simulink model "Multi_Agent_Problem"  (R2022a)
settings: Solver=ode45  StartTime=0.0  StopTime=20  RelTol=1e-3
values from neighbouring files (symbols this model uses):
  B1_inv = B1_inv(:,2)    [Dynamic_Inversion.m]    (also in Linear_Model.mat = [0.0377096774194 0 -0.0377096774194 0])
  B2_inv = B2_inv(:,2)    [Dynamic_Inversion.m]    (also in Linear_Model.mat = [0 -0.0371290322581 0 0.0371290322581])
  B3_inv = B3_inv(:,1)    [Dynamic_Inversion.m]    (also in Linear_Model.mat = [0.0031875 -0.0031875 0.0031875 -0.0031875])
  B4_inv = pinv(B4)    [Dynamic_Inversion.m]    (also in Linear_Model.mat = [-0.25 -0.25 -0.25 -0.25])
  eta = 1    [Properties_Quad.m]
  g = 9.8    [Properties_Quad.m]
  L = 0.155    [Properties_Quad.m]
  m = 4    [Controller_LQR.m]    (also in Properties_Quad.m = 1)
  mass = 0.9    [Properties_Quad.m]
  r = [ones(1,length(t))]    [Hinf_Controller_Create.m]    (also in Properties_Quad.m = 1.5)
  u_e = zeros(4,1)    [Controller_LQR.m]    (also in Dynamic_Inversion.m; Linear_Model.mat = [2.45 2.45 2.45 2.45])
  w1_in = 4    [Dynamic_Inversion.m]    (also in Linear_Model.mat)
  w1_out = 1    [Dynamic_Inversion.m]    (also in Linear_Model.mat)
  w2_in = 4    [Dynamic_Inversion.m]    (also in Linear_Model.mat)
  w2_out = 1    [Dynamic_Inversion.m]    (also in Linear_Model.mat)
  w3_in = 4    [Dynamic_Inversion.m]    (also in Linear_Model.mat)
  w4_in = 3    [Dynamic_Inversion.m]    (also in Linear_Model.mat)
  zeta1_in = 0.7    [Dynamic_Inversion.m]    (also in Linear_Model.mat)
  zeta1_out = 0.7    [Dynamic_Inversion.m]    (also in Linear_Model.mat)
  zeta2_in = 0.7    [Dynamic_Inversion.m]    (also in Linear_Model.mat)
  zeta2_out = 0.7    [Dynamic_Inversion.m]    (also in Linear_Model.mat)
  zeta3_in = 0.7    [Dynamic_Inversion.m]    (also in Linear_Model.mat)
  zeta4_in = 0.7    [Dynamic_Inversion.m]    (also in Linear_Model.mat)
undefined symbols (not defined in the file or in its folder): magnitude
libraries: aerolibutil x4, rllib x3, shared6dof x3
(part 1 of 2)
settings Model: Creator=vicen  LastModifiedBy=vicen
settings DebuggingCC: UnconnectedInputMsg=warning  UnconnectedOutputMsg=warning  UnconnectedLineMsg=warning
settings RTWCC: DLArmComputeVersion=19.05

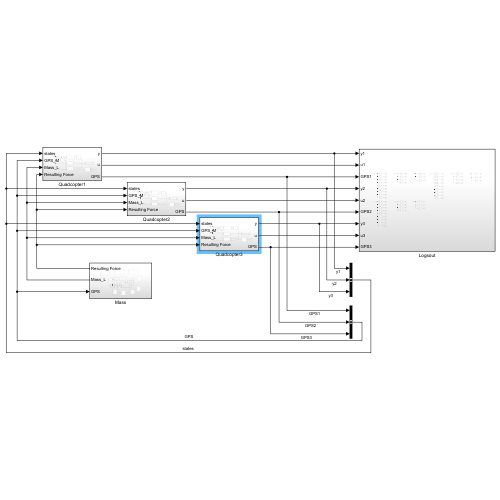
[thumbnail: Simulink's stored preview of the top-level diagram]
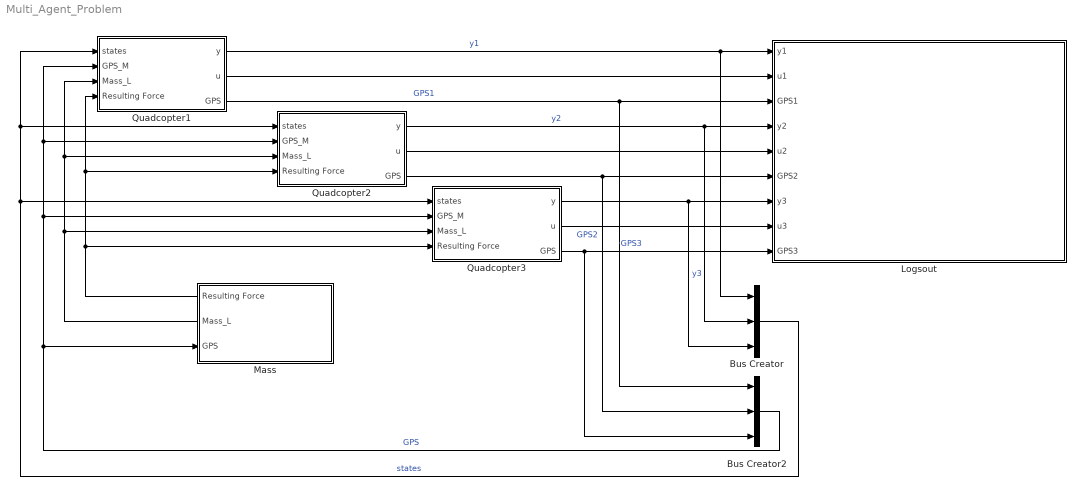
== system Multi_Agent_Problem ==
  Bus Creator : BusCreator  Inputs=3
  Bus Creator2 : BusCreator  Inputs=3
  Logsout : Subsystem
  Mass : Subsystem
      settings: PortSchema="{\"entries\":[{\"content\":{\"sides\":[{\"content\":{\"connectorIds\":[\"Out1\",\"Out2\",\"In1\"]},\"type\":\"ConnectorPlacement.EquallySpacedRectSide\",\"uuid\":\"4edc069a-805e-4b8f-97a6-cf234fccdbf6\"},{\"content\":{\"connectorIds\":[],\"side\":\"RIGHT\"},\"type\":\"ConnectorPlacement.EquallySpacedRectSide\",\"uuid\":\"8a591d16-4bf7-485b-b559-b7d05b260f63\"},{\"content\":{\"connectorIds\":[],\"side\":\"TOP\"},\"type\":\"ConnectorPlacement.EquallySpacedRectSide\",\"uuid\":\"cabdf924-e171-4e83-9a3e-1a1cf6358306\"},{\"content\":{\"connectorIds\":[],\"side\":\"BOTTOM\"},\"type\":\"ConnectorPlacement.EquallySpacedRectSide\",\"uuid\":\"5e829002-7c81-40d6-aefe-71acdfd17489\"}]},\"type\":\"ConnectorPlacement.EquallySpacedConnector\",\"uuid\":\"c7584162-5ecb-4d0e-90b3-ad9ea7690d4d\"}],\"packageUris\":[\"http://schema.mathworks.com/mf0/Connector/R2020b\"],\"version\":\"1.0\"}"
  Quadcopter1 : Subsystem
  Quadcopter2 : Subsystem
  Quadcopter3 : Subsystem
  wires:
  Quadcopter1/1(y) -> Logsout/1(y1), Bus Creator/1  "y1"
  Quadcopter1/2(u) -> Logsout/2(u1)
  Quadcopter1/3(GPS) -> Bus Creator2/1, Logsout/3(GPS1)  "GPS1"
  Quadcopter2/1(y) -> Logsout/4(y2), Bus Creator/2  "y2"
  Quadcopter2/2(u) -> Logsout/5(u2)
  Quadcopter2/3(GPS) -> Bus Creator2/2, Logsout/6(GPS2)  "GPS2"
  Quadcopter3/1(y) -> Logsout/7(y3), Bus Creator/3  "y3"
  Quadcopter3/2(u) -> Logsout/8(u3)
  Quadcopter3/3(GPS) -> Bus Creator2/3, Logsout/9(GPS3)  "GPS3"
  Bus Creator/1 -> Quadcopter3/1(states), Quadcopter2/1(states), Quadcopter1/1(states)  "states"
  Bus Creator2/1 -> Mass/1(GPS), Quadcopter3/2(GPS_M), Quadcopter2/2(GPS_M), Quadcopter1/2(GPS_M)  "GPS"
  Mass/1(Resulting Force) -> Quadcopter3/4("Resulting Force "), Quadcopter2/4("Resulting Force "), Quadcopter1/4("Resulting Force ")
  Mass/2(Mass_L) -> Quadcopter3/3(Mass_L), Quadcopter2/3(Mass_L), Quadcopter1/3(Mass_L)

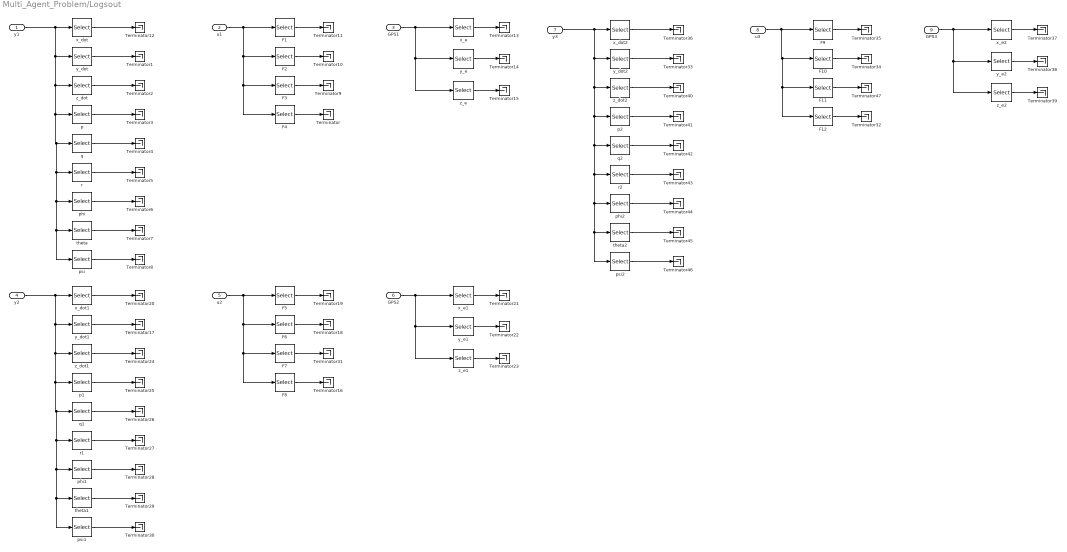
== system Multi_Agent_Problem/Logsout ==
  y1 : Inport
  u1 : Inport  Port=2
  GPS1 : Inport  Port=3
  y2 : Inport  Port=4
  u2 : Inport  Port=5
  GPS2 : Inport  Port=6
  y3 : Inport  Port=7
  u3 : Inport  Port=8
  GPS3 : Inport  Port=9
  F1 : Selector  InputPortWidth=4  IndexOptions=Index vector (dialog)  Indices=1  OutputSizes=1
  F10 : Selector  InputPortWidth=4  IndexOptions=Index vector (dialog)  Indices=2  OutputSizes=1
  F11 : Selector  InputPortWidth=4  IndexOptions=Index vector (dialog)  Indices=3  OutputSizes=1
  F12 : Selector  InputPortWidth=4  IndexOptions=Index vector (dialog)  Indices=4  OutputSizes=1
  F2 : Selector  InputPortWidth=4  IndexOptions=Index vector (dialog)  Indices=2  OutputSizes=1
  F3 : Selector  InputPortWidth=4  IndexOptions=Index vector (dialog)  Indices=3  OutputSizes=1
  F4 : Selector  InputPortWidth=4  IndexOptions=Index vector (dialog)  Indices=4  OutputSizes=1
  F5 : Selector  InputPortWidth=4  IndexOptions=Index vector (dialog)  Indices=1  OutputSizes=1
  F6 : Selector  InputPortWidth=4  IndexOptions=Index vector (dialog)  Indices=2  OutputSizes=1
  F7 : Selector  InputPortWidth=4  IndexOptions=Index vector (dialog)  Indices=3  OutputSizes=1
  F8 : Selector  InputPortWidth=4  IndexOptions=Index vector (dialog)  Indices=4  OutputSizes=1
  F9 : Selector  InputPortWidth=4  IndexOptions=Index vector (dialog)  Indices=1  OutputSizes=1
  Terminator{,1..47} (48 alike) : Terminator
  p : Selector  InputPortWidth=9  IndexOptions=Index vector (dialog)  Indices=4  OutputSizes=1
  p1 : Selector  InputPortWidth=9  IndexOptions=Index vector (dialog)  Indices=4  OutputSizes=1
  p2 : Selector  InputPortWidth=9  IndexOptions=Index vector (dialog)  Indices=4  OutputSizes=1
  phi : Selector  InputPortWidth=9  IndexOptions=Index vector (dialog)  Indices=7  OutputSizes=1
  phi1 : Selector  InputPortWidth=9  IndexOptions=Index vector (dialog)  Indices=7  OutputSizes=1
  phi2 : Selector  InputPortWidth=9  IndexOptions=Index vector (dialog)  Indices=7  OutputSizes=1
  psi : Selector  InputPortWidth=9  IndexOptions=Index vector (dialog)  Indices=9  OutputSizes=1
  psi1 : Selector  InputPortWidth=9  IndexOptions=Index vector (dialog)  Indices=9  OutputSizes=1
  psi2 : Selector  InputPortWidth=9  IndexOptions=Index vector (dialog)  Indices=9  OutputSizes=1
  q : Selector  InputPortWidth=9  IndexOptions=Index vector (dialog)  Indices=5  OutputSizes=1
  q1 : Selector  InputPortWidth=9  IndexOptions=Index vector (dialog)  Indices=5  OutputSizes=1
  q2 : Selector  InputPortWidth=9  IndexOptions=Index vector (dialog)  Indices=5  OutputSizes=1
  r : Selector  InputPortWidth=9  IndexOptions=Index vector (dialog)  Indices=6  OutputSizes=1
  r1 : Selector  InputPortWidth=9  IndexOptions=Index vector (dialog)  Indices=6  OutputSizes=1
  r2 : Selector  InputPortWidth=9  IndexOptions=Index vector (dialog)  Indices=6  OutputSizes=1
  theta : Selector  InputPortWidth=9  IndexOptions=Index vector (dialog)  Indices=8  OutputSizes=1
  theta1 : Selector  InputPortWidth=9  IndexOptions=Index vector (dialog)  Indices=8  OutputSizes=1
  theta2 : Selector  InputPortWidth=9  IndexOptions=Index vector (dialog)  Indices=8  OutputSizes=1
  x_dot : Selector  InputPortWidth=9  IndexOptions=Index vector (dialog)  Indices=1  OutputSizes=1
  x_dot1 : Selector  InputPortWidth=9  IndexOptions=Index vector (dialog)  Indices=1  OutputSizes=1
  x_dot2 : Selector  InputPortWidth=9  IndexOptions=Index vector (dialog)  Indices=1  OutputSizes=1
  x_e : Selector  InputPortWidth=3  IndexOptions=Index vector (dialog)  Indices=1  OutputSizes=1
  x_e1 : Selector  InputPortWidth=3  IndexOptions=Index vector (dialog)  Indices=1  OutputSizes=1
  x_e2 : Selector  InputPortWidth=3  IndexOptions=Index vector (dialog)  Indices=1  OutputSizes=1
  y_dot : Selector  InputPortWidth=9  IndexOptions=Index vector (dialog)  Indices=2  OutputSizes=1
  y_dot1 : Selector  InputPortWidth=9  IndexOptions=Index vector (dialog)  Indices=2  OutputSizes=1
  y_dot2 : Selector  InputPortWidth=9  IndexOptions=Index vector (dialog)  Indices=2  OutputSizes=1
  y_e : Selector  InputPortWidth=3  IndexOptions=Index vector (dialog)  Indices=2  OutputSizes=1
  y_e1 : Selector  InputPortWidth=3  IndexOptions=Index vector (dialog)  Indices=2  OutputSizes=1
  y_e2 : Selector  InputPortWidth=3  IndexOptions=Index vector (dialog)  Indices=2  OutputSizes=1
  z_dot : Selector  InputPortWidth=9  IndexOptions=Index vector (dialog)  Indices=3  OutputSizes=1
  z_dot1 : Selector  InputPortWidth=9  IndexOptions=Index vector (dialog)  Indices=3  OutputSizes=1
  z_dot2 : Selector  InputPortWidth=9  IndexOptions=Index vector (dialog)  Indices=3  OutputSizes=1
  z_e : Selector  InputPortWidth=3  IndexOptions=Index vector (dialog)  Indices=3  OutputSizes=1
  z_e1 : Selector  InputPortWidth=3  IndexOptions=Index vector (dialog)  Indices=3  OutputSizes=1
  z_e2 : Selector  InputPortWidth=3  IndexOptions=Index vector (dialog)  Indices=3  OutputSizes=1
  wires:
  y1/1 -> psi/1, theta/1, phi/1, r/1, q/1, p/1, z_dot/1, y_dot/1, x_dot/1
  x_dot/1 -> Terminator12/1
  y_dot/1 -> Terminator1/1
  z_dot/1 -> Terminator2/1
  p/1 -> Terminator3/1
  q/1 -> Terminator4/1
  r/1 -> Terminator5/1
  phi/1 -> Terminator6/1
  theta/1 -> Terminator7/1
  psi/1 -> Terminator8/1
  u1/1 -> F4/1, F3/1, F2/1, F1/1
  F1/1 -> Terminator11/1
  F2/1 -> Terminator10/1
  F3/1 -> Terminator9/1
  F4/1 -> Terminator/1
  GPS1/1 -> z_e/1, y_e/1, x_e/1
  x_e/1 -> Terminator13/1
  y_e/1 -> Terminator14/1
  z_e/1 -> Terminator15/1
  z_e1/1 -> Terminator23/1
  y_e1/1 -> Terminator22/1
  x_e1/1 -> Terminator21/1
  GPS2/1 -> x_e1/1, y_e1/1, z_e1/1
  F8/1 -> Terminator16/1
  F7/1 -> Terminator31/1
  F6/1 -> Terminator18/1
  F5/1 -> Terminator19/1
  u2/1 -> F5/1, F6/1, F7/1, F8/1
  psi1/1 -> Terminator30/1
  theta1/1 -> Terminator29/1
  phi1/1 -> Terminator28/1
  r1/1 -> Terminator27/1
  q1/1 -> Terminator26/1
  p1/1 -> Terminator25/1
  z_dot1/1 -> Terminator24/1
  y_dot1/1 -> Terminator17/1
  x_dot1/1 -> Terminator20/1
  y2/1 -> x_dot1/1, y_dot1/1, z_dot1/1, p1/1, q1/1, r1/1, phi1/1, theta1/1, psi1/1
  z_e2/1 -> Terminator39/1
  y_e2/1 -> Terminator38/1
  x_e2/1 -> Terminator37/1
  GPS3/1 -> x_e2/1, y_e2/1, z_e2/1
  F12/1 -> Terminator32/1
  F11/1 -> Terminator47/1
  F10/1 -> Terminator34/1
  F9/1 -> Terminator35/1
  u3/1 -> F9/1, F10/1, F11/1, F12/1
  psi2/1 -> Terminator46/1
  theta2/1 -> Terminator45/1
  phi2/1 -> Terminator44/1
  r2/1 -> Terminator43/1
  q2/1 -> Terminator42/1
  p2/1 -> Terminator41/1
  z_dot2/1 -> Terminator40/1
  y_dot2/1 -> Terminator33/1
  x_dot2/1 -> Terminator36/1
  y3/1 -> x_dot2/1, y_dot2/1, z_dot2/1, p2/1, q2/1, r2/1, phi2/1, theta2/1, psi2/1

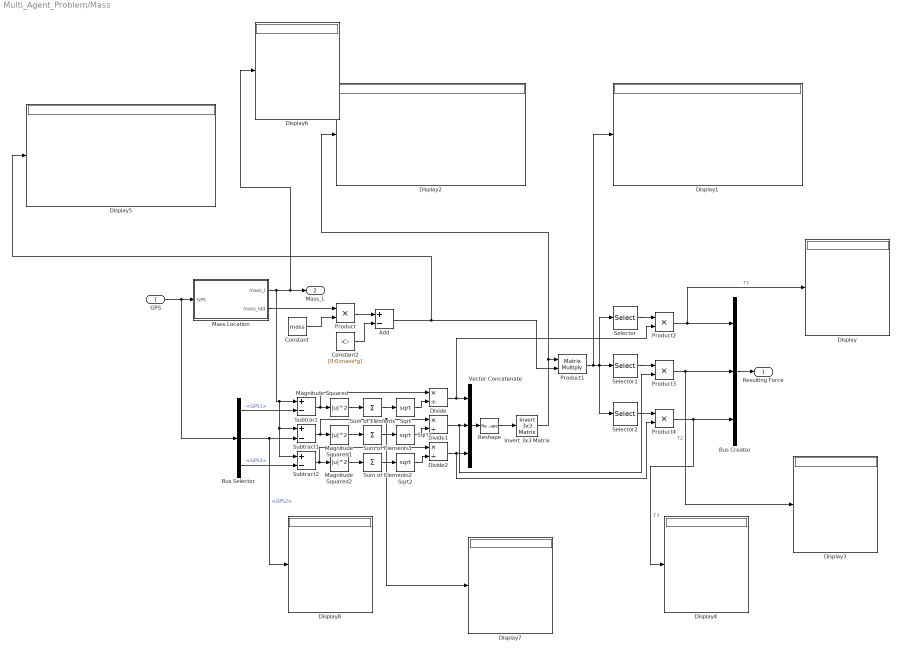
== system Multi_Agent_Problem/Mass ==
  GPS : Inport
  Add : Sum  Inputs=+-
  Bus Creator : BusCreator  Inputs=3
  Bus Selector : BusSelector  OutputSignals=GPS1,GPS2,GPS3
  Constant : Constant  Value=mass
  Constant2 : Constant  Value=[0;0;mass*g]
  Display{,1..8} (9 alike) : Display
  Divide : Product  Inputs=*/
  Divide1 : Product  Inputs=*/
  Divide2 : Product  Inputs=*/
  Invert 3x3 Matrix : aerolibutil/Invert  3x3 Matrix
  Magnitude Squared : Math  Operator=magnitude^2
  Magnitude Squared1 : Math  Operator=magnitude^2
  Magnitude Squared2 : Math  Operator=magnitude^2
  Mass Location : Subsystem
  Product{,2..4} (4 alike) : Product
  Product1 : Product  Multiplication=Matrix(*)
  Reshape : Reshape  OutputDimensionality=Customize  OutputDimensions=[3,3]
  Selector : Selector  InputPortWidth=3  IndexOptions=Index vector (dialog)  Indices=1  OutputSizes=1
  Selector1 : Selector  InputPortWidth=3  IndexOptions=Index vector (dialog)  Indices=2  OutputSizes=1
  Selector2 : Selector  InputPortWidth=3  IndexOptions=Index vector (dialog)  Indices=3  OutputSizes=1
  Sqrt : Sqrt
  Sqrt1 : Sqrt
  Sqrt2 : Sqrt
  Subtract : Sum  Inputs=+-
  Subtract1 : Sum  Inputs=+-
  Subtract2 : Sum  Inputs=+-
  Sum of Elements : Sum  Inputs=+
  Sum of Elements1 : Sum  Inputs=+
  Sum of Elements2 : Sum  Inputs=+
  Vector Concatenate : Concatenate  NumInputs=3
  Resulting Force : Outport
  Mass_L : Outport  Port=2
  wires:
  Constant/1 -> Product/2
  GPS/1 -> Bus Selector/1, Mass Location/1(GPS)
  Product/1 -> Add/1
  Constant2/1 -> Add/2
  Add/1 -> Display5/1, Product1/2
  Mass Location/2(mass_ldd) -> Product/1
  Bus Selector/1 -> Subtract/2  "<GPS1>"
  Bus Selector/2 -> Display8/1, Subtract1/2  "<GPS2>"
  Bus Selector/3 -> Subtract2/2  "<GPS3>"
  Magnitude Squared/1 -> Sum of Elements/1
  Sum of Elements/1 -> Sqrt/1
  Subtract/1 -> Divide/1, Magnitude Squared/1
  Sum of Elements1/1 -> Sqrt1/1
  Magnitude Squared1/1 -> Sum of Elements1/1
  Magnitude Squared2/1 -> Sum of Elements2/1
  Sum of Elements2/1 -> Sqrt2/1
  Subtract1/1 -> Display7/1, Divide1/1, Magnitude Squared1/1
  Subtract2/1 -> Divide2/1, Magnitude Squared2/1
  Sqrt/1 -> Divide/2
  Sqrt1/1 -> Divide1/2
  Sqrt2/1 -> Divide2/2
  Vector Concatenate/1 -> Reshape/1
  Reshape/1 -> Invert 3x3 Matrix/1
  Invert 3x3 Matrix/1 -> Display2/1, Product1/1
  Product1/1 -> Display1/1, Selector/1, Selector1/1, Selector2/1
  Selector/1 -> Product2/1
  Selector1/1 -> Product3/1
  Selector2/1 -> Product4/1
  Divide/1 -> Product2/2, Vector Concatenate/1
  Divide1/1 -> Vector Concatenate/2, Product3/2
  Divide2/1 -> Vector Concatenate/3, Product4/2
  Product2/1 -> Bus Creator/1, Display/1  "T1"
  Product3/1 -> Bus Creator/2, Display3/1  "T2"
  Product4/1 -> Bus Creator/3, Display4/1  "T3"
  Bus Creator/1 -> Resulting Force/1
  Mass Location/1(mass_l) -> Subtract1/1, Subtract2/1, Subtract/1, Display6/1, Mass_L/1

== system Multi_Agent_Problem/Quadcopter1 ==
  states : Inport
  GPS_M : Inport  Port=2
  Mass_L : Inport  Port=3
  "Resulting Force " : Inport  Port=4
  Add : Sum
  Bus Selector : BusSelector  OutputSignals=y,GPS
  Bus Selector1 : BusSelector  OutputSignals=T1
  Constant : Constant  Value=u_e
  Inner Loop Controller : Subsystem
      settings: PortSchema="{\"entries\":[{\"content\":{\"sides\":[{\"content\":{\"connectorIds\":[\"In1\"]},\"type\":\"ConnectorPlacement.EquallySpacedRectSide\",\"uuid\":\"666e7364-b111-4755-8f1d-083b40822e0a\"},{\"content\":{\"connectorIds\":[\"Out1\",\"In2\",\"In3\"],\"side\":\"RIGHT\"},\"type\":\"ConnectorPlacement.EquallySpacedRectSide\",\"uuid\":\"79960851-d5f8-4ed1-a120-baa8ff5c91cc\"},{\"content\":{\"connectorIds\":[],\"side\":\"TOP\"},\"type\":\"ConnectorPlacement.EquallySpacedRectSide\",\"uuid\":\"7e17e0c8-a495-4336-a986-2912f57e855c\"}]},\"type\":\"ConnectorPlacement.EquallySpacedConnector\",\"uuid\":\"73e8834a-8f7e-4b97-a075-5988e4100682\"}],\"packageUris\":[\"http://schema.mathworks.com/mf0/Connector/R2020b\"],\"version\":\"1.0\"}"
  Invert 3x3 Matrix : aerolibutil/Invert  3x3 Matrix
  Mission Planner : Subsystem
  Nonlinear System : Subsystem
      settings: PortSchema="{\"entries\":[{\"content\":{\"sides\":[{\"content\":{\"connectorIds\":[\"In1\",\"In2\",\"Out3\"]},\"type\":\"ConnectorPlacement.EquallySpacedRectSide\",\"uuid\":\"cab06217-b179-45bf-86f1-9cea28acaed0\"},{\"content\":{\"connectorIds\":[\"Out1\",\"Out2\"],\"side\":\"RIGHT\"},\"type\":\"ConnectorPlacement.EquallySpacedRectSide\",\"uuid\":\"5b831b23-67c9-4c45-aa0b-c8fd683f7f92\"},{\"content\":{\"connectorIds\":[],\"side\":\"TOP\"},\"type\":\"ConnectorPlacement.EquallySpacedRectSide\",\"uuid\":\"cc9770f4-03a0-4d6b-bae9-66d47aa444fc\"}]},\"type\":\"ConnectorPlacement.EquallySpacedConnector\",\"uuid\":\"fadffd99-ec6a-40bb-bf99-42c072ecc200\"}],\"packageUris\":[\"http://schema.mathworks.com/mf0/Connector/R2020b\"],\"version\":\"1.0\"}"
  Outer Loop Controller : Subsystem
      settings: PortSchema="{\"entries\":[{\"content\":{\"sides\":[{\"content\":{\"connectorIds\":[\"In1\",\"In2\"]},\"type\":\"ConnectorPlacement.EquallySpacedRectSide\",\"uuid\":\"0909ecc3-b9ee-46d0-b494-8211f486c818\"},{\"content\":{\"connectorIds\":[\"Out1\",\"In3\"],\"side\":\"RIGHT\"},\"type\":\"ConnectorPlacement.EquallySpacedRectSide\",\"uuid\":\"005e7a1d-8b7a-4f17-bab5-535ca2dfed14\"},{\"content\":{\"connectorIds\":[],\"side\":\"TOP\"},\"type\":\"ConnectorPlacement.EquallySpacedRectSide\",\"uuid\":\"0a4038b9-1305-4628-a808-cbdb517a3351\"}]},\"type\":\"ConnectorPlacement.EquallySpacedConnector\",\"uuid\":\"d0044b2e-92c2-4718-8256-3cc5618cd0b9\"}],\"packageUris\":[\"http://schema.mathworks.com/mf0/Connector/R2020b\"],\"version\":\"1.0\"}"
  Product : Product  Multiplication=Matrix(*)
  Sensors : Subsystem
  y : Outport
  u : Outport  Port=2
  GPS : Outport  Port=3
  wires:
  Nonlinear System/1(X_e) -> Sensors/1(X_e)
  Nonlinear System/2(x) -> Sensors/2(States)
  Sensors/1(Measured States) -> Inner Loop Controller/1(Measured States), Outer Loop Controller/1(Measured States), Bus Selector/1
  Outer Loop Controller/1(Outter Loop) -> Inner Loop Controller/3(Outter Loop)
  Bus Selector/2 -> GPS/1  "<GPS>"
  Bus Selector/1 -> y/1  "<y>"
  Mission Planner/1(Mission Planner) -> Outer Loop Controller/2(Mission Planner)
  Inner Loop Controller/1(u) -> Add/2
  Add/1 -> u/1, Nonlinear System/2(u)
  Constant/1 -> Add/1
  states/1 -> Mission Planner/2(states)
  GPS_M/1 -> Mission Planner/1(GPS)
  "Resulting Force "/1 -> Bus Selector1/1
  Mass_L/1 -> Mission Planner/3(Mass_L)
  Bus Selector1/1 -> Product/1, Nonlinear System/1(Resulting Force)  "<T1>"
  Nonlinear System/3(E2B) -> Invert 3x3 Matrix/1
  Invert 3x3 Matrix/1 -> Product/2
  Product/1 -> Outer Loop Controller/3(Tension Force), Inner Loop Controller/2(" Tension Force")

== system Multi_Agent_Problem/Quadcopter2 ==
  states : Inport
  GPS_M : Inport  Port=2
  Mass_L : Inport  Port=3
  "Resulting Force " : Inport  Port=4
  Add : Sum
  Bus Selector : BusSelector  OutputSignals=y,GPS
  Bus Selector1 : BusSelector  OutputSignals=T2
  Constant : Constant  Value=u_e
  Inner Loop Controller : Subsystem
      settings: PortSchema="{\"entries\":[{\"content\":{\"sides\":[{\"content\":{\"connectorIds\":[\"In1\"]},\"type\":\"ConnectorPlacement.EquallySpacedRectSide\",\"uuid\":\"666e7364-b111-4755-8f1d-083b40822e0a\"},{\"content\":{\"connectorIds\":[\"Out1\",\"In2\",\"In3\"],\"side\":\"RIGHT\"},\"type\":\"ConnectorPlacement.EquallySpacedRectSide\",\"uuid\":\"79960851-d5f8-4ed1-a120-baa8ff5c91cc\"},{\"content\":{\"connectorIds\":[],\"side\":\"TOP\"},\"type\":\"ConnectorPlacement.EquallySpacedRectSide\",\"uuid\":\"7e17e0c8-a495-4336-a986-2912f57e855c\"}]},\"type\":\"ConnectorPlacement.EquallySpacedConnector\",\"uuid\":\"73e8834a-8f7e-4b97-a075-5988e4100682\"}],\"packageUris\":[\"http://schema.mathworks.com/mf0/Connector/R2020b\"],\"version\":\"1.0\"}"
  Invert 3x3 Matrix : aerolibutil/Invert  3x3 Matrix
  Mission Planner : Subsystem
  Nonlinear System : Subsystem
      settings: PortSchema="{\"entries\":[{\"content\":{\"sides\":[{\"content\":{\"connectorIds\":[\"In1\",\"In2\",\"Out3\"]},\"type\":\"ConnectorPlacement.EquallySpacedRectSide\",\"uuid\":\"cab06217-b179-45bf-86f1-9cea28acaed0\"},{\"content\":{\"connectorIds\":[\"Out1\",\"Out2\"],\"side\":\"RIGHT\"},\"type\":\"ConnectorPlacement.EquallySpacedRectSide\",\"uuid\":\"5b831b23-67c9-4c45-aa0b-c8fd683f7f92\"},{\"content\":{\"connectorIds\":[],\"side\":\"TOP\"},\"type\":\"ConnectorPlacement.EquallySpacedRectSide\",\"uuid\":\"cc9770f4-03a0-4d6b-bae9-66d47aa444fc\"}]},\"type\":\"ConnectorPlacement.EquallySpacedConnector\",\"uuid\":\"fadffd99-ec6a-40bb-bf99-42c072ecc200\"}],\"packageUris\":[\"http://schema.mathworks.com/mf0/Connector/R2020b\"],\"version\":\"1.0\"}"
  Outer Loop Controller : Subsystem
      settings: PortSchema="{\"entries\":[{\"content\":{\"sides\":[{\"content\":{\"connectorIds\":[\"In1\",\"In2\"]},\"type\":\"ConnectorPlacement.EquallySpacedRectSide\",\"uuid\":\"0909ecc3-b9ee-46d0-b494-8211f486c818\"},{\"content\":{\"connectorIds\":[\"Out1\",\"In3\"],\"side\":\"RIGHT\"},\"type\":\"ConnectorPlacement.EquallySpacedRectSide\",\"uuid\":\"005e7a1d-8b7a-4f17-bab5-535ca2dfed14\"},{\"content\":{\"connectorIds\":[],\"side\":\"TOP\"},\"type\":\"ConnectorPlacement.EquallySpacedRectSide\",\"uuid\":\"0a4038b9-1305-4628-a808-cbdb517a3351\"}]},\"type\":\"ConnectorPlacement.EquallySpacedConnector\",\"uuid\":\"d0044b2e-92c2-4718-8256-3cc5618cd0b9\"}],\"packageUris\":[\"http://schema.mathworks.com/mf0/Connector/R2020b\"],\"version\":\"1.0\"}"
  Product : Product  Multiplication=Matrix(*)
  Sensors : Subsystem
  y : Outport
  u : Outport  Port=2
  GPS : Outport  Port=3
  wires:
  Mass_L/1 -> Mission Planner/3(Mass_L)
  "Resulting Force "/1 -> Bus Selector1/1
  GPS_M/1 -> Mission Planner/1(GPS)
  states/1 -> Mission Planner/2(states)
  Constant/1 -> Add/1
  Add/1 -> u/1, Nonlinear System/2(u)
  Inner Loop Controller/1(u) -> Add/2
  Mission Planner/1(Mission Planner) -> Outer Loop Controller/2(Mission Planner)
  Bus Selector/1 -> y/1  "<y>"
  Bus Selector/2 -> GPS/1  "<GPS>"
  Outer Loop Controller/1(Outter Loop) -> Inner Loop Controller/3(Outter Loop)
  Sensors/1(Measured States) -> Inner Loop Controller/1(Measured States), Outer Loop Controller/1(Measured States), Bus Selector/1
  Nonlinear System/2(x) -> Sensors/2(States)
  Nonlinear System/1(X_e) -> Sensors/1(X_e)
  Bus Selector1/1 -> Nonlinear System/1(Resulting Force), Product/1  "<T2>"
  Invert 3x3 Matrix/1 -> Product/2
  Product/1 -> Inner Loop Controller/2(Tension Force), Outer Loop Controller/3(Tension Force)
  Nonlinear System/3(E2B) -> Invert 3x3 Matrix/1

== system Multi_Agent_Problem/Quadcopter3 ==
  states : Inport
  GPS_M : Inport  Port=2
  Mass_L : Inport  Port=3
  "Resulting Force " : Inport  Port=4
  Add : Sum
  Bus Selector : BusSelector  OutputSignals=y,GPS
  Bus Selector1 : BusSelector  OutputSignals=T3
  Constant : Constant  Value=u_e
  Inner Loop Controller : Subsystem
      settings: PortSchema="{\"entries\":[{\"content\":{\"sides\":[{\"content\":{\"connectorIds\":[\"In1\"]},\"type\":\"ConnectorPlacement.EquallySpacedRectSide\",\"uuid\":\"666e7364-b111-4755-8f1d-083b40822e0a\"},{\"content\":{\"connectorIds\":[\"Out1\",\"In2\",\"In3\"],\"side\":\"RIGHT\"},\"type\":\"ConnectorPlacement.EquallySpacedRectSide\",\"uuid\":\"79960851-d5f8-4ed1-a120-baa8ff5c91cc\"},{\"content\":{\"connectorIds\":[],\"side\":\"TOP\"},\"type\":\"ConnectorPlacement.EquallySpacedRectSide\",\"uuid\":\"7e17e0c8-a495-4336-a986-2912f57e855c\"}]},\"type\":\"ConnectorPlacement.EquallySpacedConnector\",\"uuid\":\"73e8834a-8f7e-4b97-a075-5988e4100682\"}],\"packageUris\":[\"http://schema.mathworks.com/mf0/Connector/R2020b\"],\"version\":\"1.0\"}"
  Invert 3x3 Matrix : aerolibutil/Invert  3x3 Matrix
  Mission Planner : Subsystem
  Nonlinear System : Subsystem
      settings: PortSchema="{\"entries\":[{\"content\":{\"sides\":[{\"content\":{\"connectorIds\":[\"In1\",\"In2\",\"Out3\"]},\"type\":\"ConnectorPlacement.EquallySpacedRectSide\",\"uuid\":\"cab06217-b179-45bf-86f1-9cea28acaed0\"},{\"content\":{\"connectorIds\":[\"Out1\",\"Out2\"],\"side\":\"RIGHT\"},\"type\":\"ConnectorPlacement.EquallySpacedRectSide\",\"uuid\":\"5b831b23-67c9-4c45-aa0b-c8fd683f7f92\"},{\"content\":{\"connectorIds\":[],\"side\":\"TOP\"},\"type\":\"ConnectorPlacement.EquallySpacedRectSide\",\"uuid\":\"cc9770f4-03a0-4d6b-bae9-66d47aa444fc\"}]},\"type\":\"ConnectorPlacement.EquallySpacedConnector\",\"uuid\":\"fadffd99-ec6a-40bb-bf99-42c072ecc200\"}],\"packageUris\":[\"http://schema.mathworks.com/mf0/Connector/R2020b\"],\"version\":\"1.0\"}"
  Outer Loop Controller : Subsystem
      settings: PortSchema="{\"entries\":[{\"content\":{\"sides\":[{\"content\":{\"connectorIds\":[\"In1\",\"In2\"]},\"type\":\"ConnectorPlacement.EquallySpacedRectSide\",\"uuid\":\"0909ecc3-b9ee-46d0-b494-8211f486c818\"},{\"content\":{\"connectorIds\":[\"Out1\",\"In3\"],\"side\":\"RIGHT\"},\"type\":\"ConnectorPlacement.EquallySpacedRectSide\",\"uuid\":\"005e7a1d-8b7a-4f17-bab5-535ca2dfed14\"},{\"content\":{\"connectorIds\":[],\"side\":\"TOP\"},\"type\":\"ConnectorPlacement.EquallySpacedRectSide\",\"uuid\":\"0a4038b9-1305-4628-a808-cbdb517a3351\"}]},\"type\":\"ConnectorPlacement.EquallySpacedConnector\",\"uuid\":\"d0044b2e-92c2-4718-8256-3cc5618cd0b9\"}],\"packageUris\":[\"http://schema.mathworks.com/mf0/Connector/R2020b\"],\"version\":\"1.0\"}"
  Product : Product  Multiplication=Matrix(*)
  Sensors : Subsystem
  y : Outport
  u : Outport  Port=2
  GPS : Outport  Port=3
  wires:
  Nonlinear System/1(X_e) -> Sensors/1(X_e)
  Nonlinear System/2(x) -> Sensors/2(States)
  Sensors/1(Measured States) -> Bus Selector/1, Outer Loop Controller/1(Measured States), Inner Loop Controller/1(Measured States)
  Outer Loop Controller/1(Outter Loop) -> Inner Loop Controller/3(Outter Loop)
  Bus Selector/2 -> GPS/1  "<GPS>"
  Bus Selector/1 -> y/1  "<y>"
  Mission Planner/1(Mission Planner) -> Outer Loop Controller/2(Mission Planner)
  Inner Loop Controller/1(u) -> Add/2
  Add/1 -> u/1, Nonlinear System/2(u)
  Constant/1 -> Add/1
  states/1 -> Mission Planner/2(states)
  GPS_M/1 -> Mission Planner/1(GPS)
  "Resulting Force "/1 -> Bus Selector1/1
  Mass_L/1 -> Mission Planner/3(Mass_L)
  Bus Selector1/1 -> Nonlinear System/1(Resulting Force), Product/1  "<T3>"
  Invert 3x3 Matrix/1 -> Product/2
  Product/1 -> Outer Loop Controller/3(Tension Force), Inner Loop Controller/2(Tension Force)
  Nonlinear System/3(E2B) -> Invert 3x3 Matrix/1

== system Multi_Agent_Problem/Mass/Mass Location ==
  GPS : Inport
  Bus Selector : BusSelector  OutputSignals=GPS1,GPS2,GPS3
  Constant : Constant  Value=r
  Derivative : Derivative
  Derivative1 : Derivative
  Display{,1..4} (5 alike) : Display
  Mass Location : MATLAB Function  TreatAsAtomicUnit=on
  mass_l : Outport
  mass_ldd : Outport  Port=2
  wires:
  Constant/1 -> Display4/1, Mass Location/4(r)
  Bus Selector/3 -> Mass Location/3(P3), Display3/1  "<GPS3>"
  Bus Selector/2 -> Mass Location/2(P2), Display2/1  "<GPS2>"
  Bus Selector/1 -> Display1/1, Mass Location/1(P1)  "<GPS1>"
  GPS/1 -> Bus Selector/1
  Derivative/1 -> mass_ldd/1
  Mass Location/1(mass_l) -> Display/1, mass_l/1, Derivative1/1
  Derivative1/1 -> Derivative/1

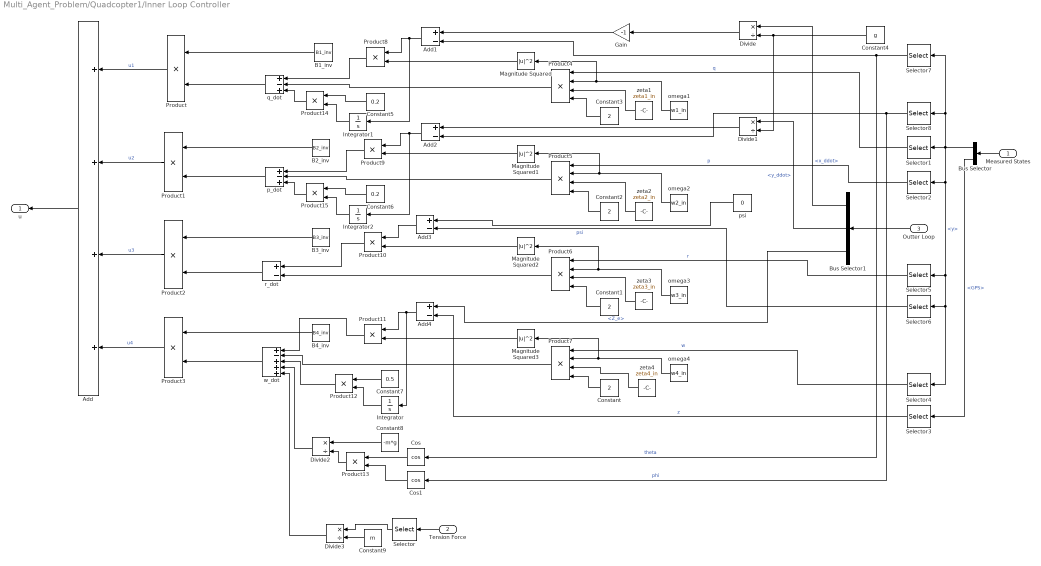
== system Multi_Agent_Problem/Quadcopter1/Inner Loop Controller ==
  Measured States : Inport
  " Tension Force" : Inport  Port=2
  Outter Loop : Inport  Port=3
  Add : Sum  Inputs=++++
  Add{1..4} (4 alike) : Sum  Inputs=+-
  B1_inv : Constant  Value=B1_inv
  B2_inv : Constant  Value=B2_inv
  B3_inv : Constant  Value=B3_inv
  B4_inv : Constant  Value=B4_inv
  Bus Selector : BusSelector  OutputSignals=y,GPS
  Bus Selector1 : BusSelector  OutputSignals=x_ddot,y_ddot,Z_e
  Constant{,1..3} (4 alike) : Constant  Value=2
  Constant4 : Constant  Value=g
  Constant5 : Constant  Value=0.2
  Constant6 : Constant  Value=0.2
  Constant7 : Constant  Value=0.5
  Constant8 : Constant  Value=-m*g
  Constant9 : Constant  Value=m
  Cos : Trigonometry  Operator=cos
  Cos1 : Trigonometry  Operator=cos
  Divide{,1..3} (4 alike) : Product  Inputs=*/
  Gain : Gain  Gain=-1
  Integrator : Integrator
  Integrator1 : Integrator
  Integrator2 : Integrator
  Magnitude Squared{,1..3} (4 alike) : Math  Operator=magnitude^2
  Product{,1..3,8..15} (12 alike) : Product
  Product{4..7} (4 alike) : Product  Inputs=4
  Selector : Selector  InputPortWidth=3  IndexOptions=Index vector (dialog)  Indices=3  OutputSizes=1
  Selector1 : Selector  InputPortWidth=9  IndexOptions=Index vector (dialog)  Indices=5  OutputSizes=1
  Selector2 : Selector  InputPortWidth=9  IndexOptions=Index vector (dialog)  Indices=4  OutputSizes=1
  Selector3 : Selector  InputPortWidth=3  IndexOptions=Index vector (dialog)  Indices=3  OutputSizes=1
  Selector4 : Selector  InputPortWidth=9  IndexOptions=Index vector (dialog)  Indices=3  OutputSizes=1
  Selector5 : Selector  InputPortWidth=9  IndexOptions=Index vector (dialog)  Indices=6  OutputSizes=1
  Selector6 : Selector  InputPortWidth=9  IndexOptions=Index vector (dialog)  Indices=9  OutputSizes=1
  Selector7 : Selector  InputPortWidth=9  IndexOptions=Index vector (dialog)  Indices=8  OutputSizes=1
  Selector8 : Selector  InputPortWidth=9  IndexOptions=Index vector (dialog)  Indices=7  OutputSizes=1
  omega1 : Constant  Value=w1_in
  omega2 : Constant  Value=w2_in
  omega3 : Constant  Value=w3_in
  omega4 : Constant  Value=w4_in
  p_dot : Sum  Inputs=+-+
  psi : Constant  Value=0
  q_dot : Sum  Inputs=+-+
  r_dot : Sum  Inputs=+-
  w_dot : Sum  Inputs=+-+++
  zeta1 : Constant  Value=zeta1_in
  zeta2 : Constant  Value=zeta2_in
  zeta3 : Constant  Value=zeta3_in
  zeta4 : Constant  Value=zeta4_in
  u : Outport
  wires:
  Add/1 -> u/1
  Product/1 -> Add/1  "u1"
  Product1/1 -> Add/2  "u2"
  Product2/1 -> Add/3  "u3"
  Product3/1 -> Add/4  "u4"
  B1_inv/1 -> Product/1
  B2_inv/1 -> Product1/1
  B3_inv/1 -> Product2/1
  B4_inv/1 -> Product3/1
  q_dot/1 -> Product/2
  p_dot/1 -> Product1/2
  r_dot/1 -> Product2/2
  w_dot/1 -> Product3/2
  Product8/1 -> q_dot/1
  Product9/1 -> p_dot/1
  Product10/1 -> r_dot/1
  Product11/1 -> w_dot/1
  Product4/1 -> q_dot/2
  Product5/1 -> p_dot/2
  Product6/1 -> r_dot/2
  Product7/1 -> w_dot/2
  Magnitude Squared/1 -> Product8/2
  Magnitude Squared1/1 -> Product9/2
  Magnitude Squared2/1 -> Product10/2
  Magnitude Squared3/1 -> Product11/2
  Constant/1 -> Product7/4
  Constant1/1 -> Product6/4
  Constant2/1 -> Product5/4
  Constant3/1 -> Product4/4
  zeta1/1 -> Product4/3
  zeta2/1 -> Product5/3
  zeta3/1 -> Product6/3
  omega1/1 -> Magnitude Squared/1, Product4/2
  omega2/1 -> Magnitude Squared1/1, Product5/2
  omega3/1 -> Magnitude Squared2/1, Product6/2
  omega4/1 -> Magnitude Squared3/1, Product7/2
  Measured States/1 -> Bus Selector/1
  Selector1/1 -> Product4/1  "q"
  Selector2/1 -> Product5/1  "p"
  Selector5/1 -> Product6/1  "r"
  Selector4/1 -> Product7/1  "w"
  zeta4/1 -> Product7/3
  Add3/1 -> Product10/1
  Add4/1 -> Integrator/1, Product11/1
  Outter Loop/1 -> Bus Selector1/1
  Bus Selector1/1 -> Divide/1  "<x_ddot>"
  Bus Selector1/2 -> Divide1/1  "<y_ddot>"
  psi/1 -> Add3/1
  Bus Selector1/3 -> Add4/1  "<Z_e>"
  Bus Selector/1 -> Selector5/1, Selector6/1, Selector4/1, Selector2/1, Selector1/1, Selector8/1, Selector7/1  "<y>"
  Divide/1 -> Gain/1
  Constant4/1 -> Divide1/2, Divide/2
  Bus Selector/2 -> Selector3/1  "<GPS>"
  Selector3/1 -> Add4/2  "z"
  Selector6/1 -> Add3/2  "psi"
  Selector8/1 -> Cos1/1, Add2/2  "phi"
  Selector7/1 -> Cos/1, Add1/2  "theta"
  Gain/1 -> Add1/1
  Divide1/1 -> Add2/1
  Constant7/1 -> Product12/1
  Integrator/1 -> Product12/2
  Product12/1 -> w_dot/3
  Cos/1 -> Product13/1
  Cos1/1 -> Product13/2
  Constant8/1 -> Divide2/1
  Product13/1 -> Divide2/2
  Divide2/1 -> w_dot/4
  Integrator1/1 -> Product14/2
  Add1/1 -> Integrator1/1, Product8/1
  Product14/1 -> q_dot/3
  Constant5/1 -> Product14/1
  Constant6/1 -> Product15/1
  Product15/1 -> p_dot/3
  Add2/1 -> Integrator2/1, Product9/1
  Integrator2/1 -> Product15/2
  " Tension Force"/1 -> Selector/1
  Constant9/1 -> Divide3/2
  Selector/1 -> Divide3/1
  Divide3/1 -> w_dot/5

== system Multi_Agent_Problem/Quadcopter1/Mission Planner ==
  GPS : Inport
  states : Inport  Port=2
  Mass_L : Inport  Port=3
  Build Observation Vector : Subsystem
  Bus Creator : BusCreator  Inputs=3
  Bus Creator1 : BusCreator  Inputs=3
  Bus Selector : BusSelector  OutputSignals=GPS1,GPS2,GPS3
  Constant : Constant  Value=3
  Constant2 : Constant  Value=-1
  Constant3 : Constant  Value=(1 + sqrt(2))
  Demux : Demux  Outputs=3
  Find Reward : MATLAB Function  TreatAsAtomicUnit=on
  RL Agent1 : rllib/RL Agent  Agent=agent1  ExternalActionAsInput=off  ProvideLastAction=off  ProvideCumRwd=off  TreatAsDirectFeedthrough=on  UseStrictObservationDataTypes=off
  Terminator : Terminator
  Mission Planner : Outport
  wires:
  Constant/1 -> Bus Creator/1  "x_e"
  Constant2/1 -> Bus Creator/2  "y_e"
  Constant3/1 -> Bus Creator/3  "h_e"
  GPS/1 -> Bus Selector/1, Build Observation Vector/2(GPS)
  Find Reward/1(reward) -> RL Agent1/2
  Find Reward/2(isdone) -> RL Agent1/3
  states/1 -> Build Observation Vector/1(states)
  Build Observation Vector/1(Obsv) -> RL Agent1/1
  RL Agent1/1 -> Demux/1
  Demux/1 -> Bus Creator1/1  "x_e"
  Demux/2 -> Bus Creator1/2  "y_e"
  Demux/3 -> Bus Creator1/3  "h_e"
  Bus Creator1/1 -> Terminator/1
  Bus Selector/1 -> Find Reward/1(GPS1)  "<GPS1>"
  Bus Selector/2 -> Find Reward/2(GPS2)  "<GPS2>"
  Bus Selector/3 -> Find Reward/3(GPS3)  "<GPS3>"
  Mass_L/1 -> Build Observation Vector/3(mass_l), Find Reward/4(GPS4)
  Bus Creator/1 -> Mission Planner/1

== system Multi_Agent_Problem/Quadcopter1/Nonlinear System ==
  Resulting Force : Inport
  u : Inport  Port=2
  6DOF (Euler Angles) : shared6dof/6DOF (Euler Angles)  units=Metric (MKS)  mtype=Fixed  rep=Euler Angles  xme_0=init_1.pos_e  Vm_0=init_1.vel_b  eul_0=init_1.Euler  pm_0=init_1.rotation_rates_b  mass_0=m  mass_e=0.5  mass_f=2.0  inertia=I  inertia_e=eye(3)  inertia_f=2*eye(3)  k_quat=1.0  vre_flag=on  abi_flag=off  aMode=0  xme_statename=''  Vm_statename=''  eul_statename=''  quat_statename=''  pm_statename=''  mass_statename=''
      settings: SourceProductBaseCode=AE,PW,DR,MT,VE
  Add : Sum
  Matrix Concatenate : Concatenate  NumInputs=3  ConcatenateDimension=2
  Product : Product  Multiplication=Matrix(*)
  Solve for Forces : Subsystem
  Solve for Moments : Subsystem
  Terminator1 : Terminator
  Terminator2 : Terminator
  Terminator3 : Terminator
  X_e : Outport
  x : Outport  Port=2
  E2B : Outport  Port=3
  wires:
  6DOF (Euler Angles)/8 -> Terminator3/1
  6DOF (Euler Angles)/1 -> Matrix Concatenate/1
  6DOF (Euler Angles)/7 -> Terminator2/1
  u/1 -> Solve for Moments/1(u), Solve for Forces/2(u)
  6DOF (Euler Angles)/6 -> Matrix Concatenate/2
  6DOF (Euler Angles)/3 -> Matrix Concatenate/3
  6DOF (Euler Angles)/5 -> Terminator1/1
  Solve for Forces/1(Forces) -> Add/2
  Solve for Moments/1(Moments) -> 6DOF (Euler Angles)/2
  6DOF (Euler Angles)/2 -> X_e/1
  Matrix Concatenate/1 -> x/1
  Resulting Force/1 -> Product/2
  Add/1 -> 6DOF (Euler Angles)/1
  Product/1 -> Add/1
  6DOF (Euler Angles)/4 -> E2B/1, Solve for Forces/1(E2B), Product/1

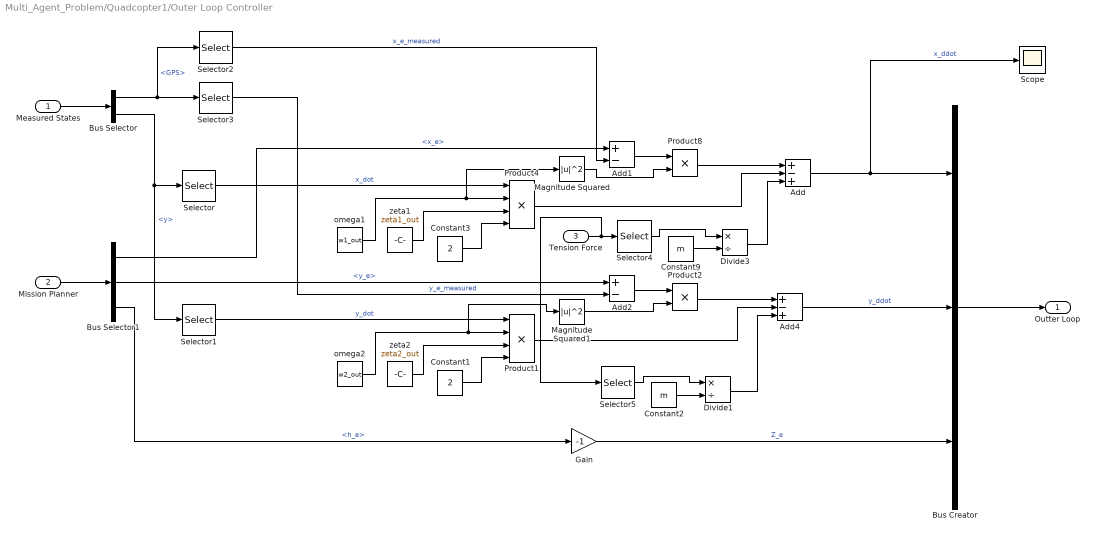
== system Multi_Agent_Problem/Quadcopter1/Outer Loop Controller ==
  Measured States : Inport
  Mission Planner : Inport  Port=2
  Tension Force : Inport  Port=3
  Add : Sum  Inputs=+-+
  Add1 : Sum  Inputs=+-
  Add2 : Sum  Inputs=+-
  Add4 : Sum  Inputs=+-+
  Bus Creator : BusCreator  Inputs=3
  Bus Selector : BusSelector  OutputSignals=GPS,y
  Bus Selector1 : BusSelector  OutputSignals=x_e,y_e,h_e
  Constant1 : Constant  Value=2
  Constant2 : Constant  Value=m
  Constant3 : Constant  Value=2
  Constant9 : Constant  Value=m
  Divide1 : Product  Inputs=*/
  Divide3 : Product  Inputs=*/
  Gain : Gain  Gain=-1
  Magnitude Squared : Math  Operator=magnitude^2
  Magnitude Squared1 : Math  Operator=magnitude^2
  Product1 : Product  Inputs=4
  Product2 : Product
  Product4 : Product  Inputs=4
  Product8 : Product
  Scope : Scope
  Selector : Selector  InputPortWidth=9  IndexOptions=Index vector (dialog)  Indices=1  OutputSizes=1
  Selector1 : Selector  InputPortWidth=9  IndexOptions=Index vector (dialog)  Indices=2  OutputSizes=1
  Selector2 : Selector  InputPortWidth=3  IndexOptions=Index vector (dialog)  Indices=1  OutputSizes=1
  Selector3 : Selector  InputPortWidth=3  IndexOptions=Index vector (dialog)  Indices=2  OutputSizes=1
  Selector4 : Selector  InputPortWidth=3  IndexOptions=Index vector (dialog)  Indices=1  OutputSizes=1
  Selector5 : Selector  InputPortWidth=3  IndexOptions=Index vector (dialog)  Indices=2  OutputSizes=1
  omega1 : Constant  Value=w1_out
  omega2 : Constant  Value=w2_out
  zeta1 : Constant  Value=zeta1_out
  zeta2 : Constant  Value=zeta2_out
  Outter Loop : Outport
  wires:
  Measured States/1 -> Bus Selector/1
  Selector/1 -> Product4/1  "x_dot"
  Product4/1 -> Add/2
  omega1/1 -> Magnitude Squared/1, Product4/2
  Bus Selector1/1 -> Add1/1  "<x_e>"
  Constant3/1 -> Product4/4
  Add1/1 -> Product8/1
  Add/1 -> Scope/1, Bus Creator/1  "x_ddot"
  zeta1/1 -> Product4/3
  Magnitude Squared/1 -> Product8/2
  Bus Creator/1 -> Outter Loop/1
  Mission Planner/1 -> Bus Selector1/1
  Bus Selector1/2 -> Add2/1  "<y_e>"
  Bus Selector/1 -> Selector3/1, Selector2/1  "<GPS>"
  Bus Selector/2 -> Selector1/1, Selector/1  "<y>"
  Selector2/1 -> Add1/2  "x_e_measured"
  Selector3/1 -> Add2/2  "y_e_measured"
  Magnitude Squared1/1 -> Product2/2
  zeta2/1 -> Product1/3
  Add4/1 -> Bus Creator/2  "y_ddot"
  Add2/1 -> Product2/1
  Constant1/1 -> Product1/4
  omega2/1 -> Magnitude Squared1/1, Product1/2
  Product1/1 -> Add4/2
  Product8/1 -> Add/1
  Product2/1 -> Add4/1
  Selector1/1 -> Product1/1  "y_dot"
  Bus Selector1/3 -> Gain/1  "<h_e>"
  Gain/1 -> Bus Creator/3  "Z_e"
  Constant9/1 -> Divide3/2
  Selector4/1 -> Divide3/1
  Tension Force/1 -> Selector5/1, Selector4/1
  Divide3/1 -> Add/3
  Divide1/1 -> Add4/3
  Constant2/1 -> Divide1/2
  Selector5/1 -> Divide1/1

== system Multi_Agent_Problem/Quadcopter1/Sensors ==
  X_e : Inport
  States : Inport  Port=2
  Bus Creator : BusCreator  Inputs=2
  Measured States : Outport
  wires:
  States/1 -> Bus Creator/2  "y"
  Bus Creator/1 -> Measured States/1
  X_e/1 -> Bus Creator/1  "GPS"

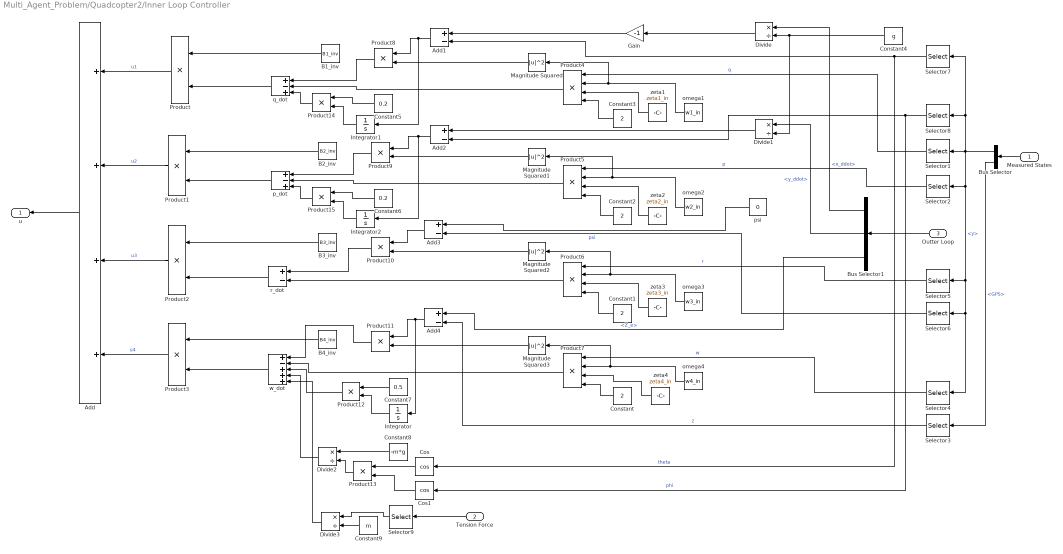
== system Multi_Agent_Problem/Quadcopter2/Inner Loop Controller ==
  Measured States : Inport
  Tension Force : Inport  Port=2
  Outter Loop : Inport  Port=3
  Add : Sum  Inputs=++++
  Add{1..4} (4 alike) : Sum  Inputs=+-
  B1_inv : Constant  Value=B1_inv
  B2_inv : Constant  Value=B2_inv
  B3_inv : Constant  Value=B3_inv
  B4_inv : Constant  Value=B4_inv
  Bus Selector : BusSelector  OutputSignals=y,GPS
  Bus Selector1 : BusSelector  OutputSignals=x_ddot,y_ddot,Z_e
  Constant{,1..3} (4 alike) : Constant  Value=2
  Constant4 : Constant  Value=g
  Constant5 : Constant  Value=0.2
  Constant6 : Constant  Value=0.2
  Constant7 : Constant  Value=0.5
  Constant8 : Constant  Value=-m*g
  Constant9 : Constant  Value=m
  Cos : Trigonometry  Operator=cos
  Cos1 : Trigonometry  Operator=cos
  Divide{,1..3} (4 alike) : Product  Inputs=*/
  Gain : Gain  Gain=-1
  Integrator : Integrator
  Integrator1 : Integrator
  Integrator2 : Integrator
  Magnitude Squared{,1..3} (4 alike) : Math  Operator=magnitude^2
  Product{,1..3,8..15} (12 alike) : Product
  Product{4..7} (4 alike) : Product  Inputs=4
  Selector1 : Selector  InputPortWidth=9  IndexOptions=Index vector (dialog)  Indices=5  OutputSizes=1
  Selector2 : Selector  InputPortWidth=9  IndexOptions=Index vector (dialog)  Indices=4  OutputSizes=1
  Selector3 : Selector  InputPortWidth=3  IndexOptions=Index vector (dialog)  Indices=3  OutputSizes=1
  Selector4 : Selector  InputPortWidth=9  IndexOptions=Index vector (dialog)  Indices=3  OutputSizes=1
  Selector5 : Selector  InputPortWidth=9  IndexOptions=Index vector (dialog)  Indices=6  OutputSizes=1
  Selector6 : Selector  InputPortWidth=9  IndexOptions=Index vector (dialog)  Indices=9  OutputSizes=1
  Selector7 : Selector  InputPortWidth=9  IndexOptions=Index vector (dialog)  Indices=8  OutputSizes=1
  Selector8 : Selector  InputPortWidth=9  IndexOptions=Index vector (dialog)  Indices=7  OutputSizes=1
  Selector9 : Selector  InputPortWidth=3  IndexOptions=Index vector (dialog)  Indices=3  OutputSizes=1
  omega1 : Constant  Value=w1_in
  omega2 : Constant  Value=w2_in
  omega3 : Constant  Value=w3_in
  omega4 : Constant  Value=w4_in
  p_dot : Sum  Inputs=+-+
  psi : Constant  Value=0
  q_dot : Sum  Inputs=+-+
  r_dot : Sum  Inputs=+-
  w_dot : Sum  Inputs=+-+++
  zeta1 : Constant  Value=zeta1_in
  zeta2 : Constant  Value=zeta2_in
  zeta3 : Constant  Value=zeta3_in
  zeta4 : Constant  Value=zeta4_in
  u : Outport
  wires:
  Integrator2/1 -> Product15/2
  Add2/1 -> Product9/1, Integrator2/1
  Product15/1 -> p_dot/3
  Constant6/1 -> Product15/1
  Constant5/1 -> Product14/1
  Product14/1 -> q_dot/3
  Add1/1 -> Product8/1, Integrator1/1
  Integrator1/1 -> Product14/2
  Divide2/1 -> w_dot/4
  Product13/1 -> Divide2/2
  Constant8/1 -> Divide2/1
  Cos1/1 -> Product13/2
  Cos/1 -> Product13/1
  Product12/1 -> w_dot/3
  Integrator/1 -> Product12/2
  Constant7/1 -> Product12/1
  Divide1/1 -> Add2/1
  Gain/1 -> Add1/1
  Selector7/1 -> Add1/2, Cos/1  "theta"
  Selector8/1 -> Add2/2, Cos1/1  "phi"
  Selector6/1 -> Add3/2  "psi"
  Selector3/1 -> Add4/2  "z"
  Bus Selector/2 -> Selector3/1  "<GPS>"
  Constant4/1 -> Divide/2, Divide1/2
  Divide/1 -> Gain/1
  Bus Selector/1 -> Selector7/1, Selector8/1, Selector1/1, Selector2/1, Selector4/1, Selector6/1, Selector5/1  "<y>"
  Bus Selector1/3 -> Add4/1  "<Z_e>"
  psi/1 -> Add3/1
  Bus Selector1/2 -> Divide1/1  "<y_ddot>"
  Bus Selector1/1 -> Divide/1  "<x_ddot>"
  Outter Loop/1 -> Bus Selector1/1
  Add4/1 -> Product11/1, Integrator/1
  Add3/1 -> Product10/1
  zeta4/1 -> Product7/3
  Selector4/1 -> Product7/1  "w"
  Selector5/1 -> Product6/1  "r"
  Selector2/1 -> Product5/1  "p"
  Selector1/1 -> Product4/1  "q"
  Measured States/1 -> Bus Selector/1
  omega4/1 -> Product7/2, Magnitude Squared3/1
  omega3/1 -> Product6/2, Magnitude Squared2/1
  omega2/1 -> Product5/2, Magnitude Squared1/1
  omega1/1 -> Product4/2, Magnitude Squared/1
  zeta3/1 -> Product6/3
  zeta2/1 -> Product5/3
  zeta1/1 -> Product4/3
  Constant3/1 -> Product4/4
  Constant2/1 -> Product5/4
  Constant1/1 -> Product6/4
  Constant/1 -> Product7/4
  Magnitude Squared3/1 -> Product11/2
  Magnitude Squared2/1 -> Product10/2
  Magnitude Squared1/1 -> Product9/2
  Magnitude Squared/1 -> Product8/2
  Product7/1 -> w_dot/2
  Product6/1 -> r_dot/2
  Product5/1 -> p_dot/2
  Product4/1 -> q_dot/2
  Product11/1 -> w_dot/1
  Product10/1 -> r_dot/1
  Product9/1 -> p_dot/1
  Product8/1 -> q_dot/1
  w_dot/1 -> Product3/2
  r_dot/1 -> Product2/2
  p_dot/1 -> Product1/2
  q_dot/1 -> Product/2
  B4_inv/1 -> Product3/1
  B3_inv/1 -> Product2/1
  B2_inv/1 -> Product1/1
  B1_inv/1 -> Product/1
  Product3/1 -> Add/4  "u4"
  Product2/1 -> Add/3  "u3"
  Product1/1 -> Add/2  "u2"
  Product/1 -> Add/1  "u1"
  Add/1 -> u/1
  Divide3/1 -> w_dot/5
  Constant9/1 -> Divide3/2
  Selector9/1 -> Divide3/1
  Tension Force/1 -> Selector9/1

== system Multi_Agent_Problem/Quadcopter2/Mission Planner ==
  GPS : Inport
  states : Inport  Port=2
  Mass_L : Inport  Port=3
  Build Observation Vector : Subsystem
  Bus Creator : BusCreator  Inputs=3
  Bus Creator1 : BusCreator  Inputs=3
  Bus Selector : BusSelector  OutputSignals=GPS1,GPS2,GPS3
  Constant : Constant  Value=2
  Constant2 : Constant  Value=-1.25
  Constant3 : Constant  Value=(1 + sqrt(1.25))
  Demux : Demux  Outputs=3
  Find Reward : MATLAB Function  TreatAsAtomicUnit=on
  RL Agent2 : rllib/RL Agent  Agent=agent2  ExternalActionAsInput=off  ProvideLastAction=off  ProvideCumRwd=off  TreatAsDirectFeedthrough=on  UseStrictObservationDataTypes=off
  Terminator : Terminator
  Mission Planner : Outport
  wires:
  Mass_L/1 -> Find Reward/4(GPS4), Build Observation Vector/3(mass_l)
  Bus Selector/3 -> Find Reward/3(GPS3)  "<GPS3>"
  Bus Selector/2 -> Find Reward/2(GPS2)  "<GPS2>"
  Bus Selector/1 -> Find Reward/1(GPS1)  "<GPS1>"
  Bus Creator1/1 -> Terminator/1
  Demux/3 -> Bus Creator1/3  "z_e"
  Demux/2 -> Bus Creator1/2  "y_e"
  Demux/1 -> Bus Creator1/1  "x_e"
  RL Agent2/1 -> Demux/1
  Build Observation Vector/1(Obsv) -> RL Agent2/1
  states/1 -> Build Observation Vector/1(states)
  Find Reward/2(isdone) -> RL Agent2/3
  Find Reward/1(reward) -> RL Agent2/2
  GPS/1 -> Build Observation Vector/2(GPS), Bus Selector/1
  Constant3/1 -> Bus Creator/3  "h_e"
  Constant2/1 -> Bus Creator/2  "y_e"
  Constant/1 -> Bus Creator/1  "x_e"
  Bus Creator/1 -> Mission Planner/1

== system Multi_Agent_Problem/Quadcopter2/Nonlinear System ==
  Resulting Force : Inport
  u : Inport  Port=2
  6DOF (Euler Angles) : shared6dof/6DOF (Euler Angles)  units=Metric (MKS)  mtype=Fixed  rep=Euler Angles  xme_0=init_2.pos_e  Vm_0=init_2.vel_b  eul_0=init_2.Euler  pm_0=init_2.rotation_rates_b  mass_0=m  mass_e=0.5  mass_f=2.0  inertia=I  inertia_e=eye(3)  inertia_f=2*eye(3)  k_quat=1.0  vre_flag=on  abi_flag=off  aMode=0  xme_statename=''  Vm_statename=''  eul_statename=''  quat_statename=''  pm_statename=''  mass_statename=''
      settings: SourceProductBaseCode=AE,PW,DR,MT,VE
  Add : Sum
  Display : Display
  Matrix Concatenate : Concatenate  NumInputs=3  ConcatenateDimension=2
  Product : Product  Multiplication=Matrix(*)
  Solve for Forces : Subsystem
  Solve for Moments : Subsystem
  Terminator1 : Terminator
  Terminator2 : Terminator
  Terminator3 : Terminator
  X_e : Outport
  x : Outport  Port=2
  E2B : Outport  Port=3
  wires:
  Resulting Force/1 -> Product/2
  Matrix Concatenate/1 -> x/1
  6DOF (Euler Angles)/2 -> X_e/1
  Solve for Moments/1(Moments) -> 6DOF (Euler Angles)/2
  Solve for Forces/1(Forces) -> Add/2
  6DOF (Euler Angles)/4 -> Product/1, E2B/1, Solve for Forces/1(E2B)
  6DOF (Euler Angles)/5 -> Terminator1/1
  6DOF (Euler Angles)/3 -> Matrix Concatenate/3
  6DOF (Euler Angles)/6 -> Matrix Concatenate/2
  u/1 -> Solve for Forces/2(u), Solve for Moments/1(u)
  6DOF (Euler Angles)/7 -> Terminator2/1
  6DOF (Euler Angles)/1 -> Matrix Concatenate/1
  6DOF (Euler Angles)/8 -> Terminator3/1
  Add/1 -> Display/1, 6DOF (Euler Angles)/1
  Product/1 -> Add/1

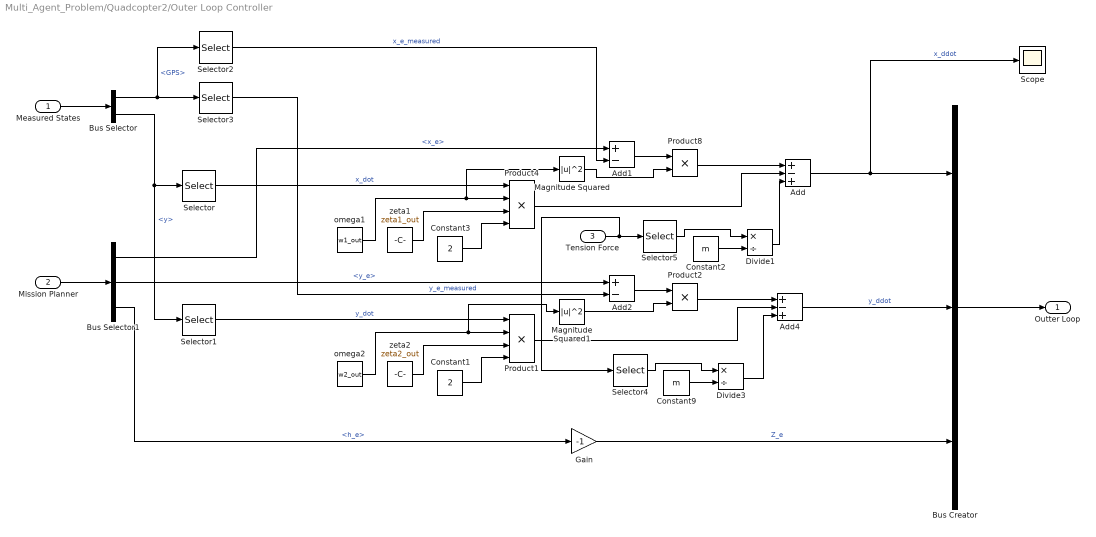
== system Multi_Agent_Problem/Quadcopter2/Outer Loop Controller ==
  Measured States : Inport
  Mission Planner : Inport  Port=2
  Tension Force : Inport  Port=3
  Add : Sum  Inputs=+-+
  Add1 : Sum  Inputs=+-
  Add2 : Sum  Inputs=+-
  Add4 : Sum  Inputs=+-+
  Bus Creator : BusCreator  Inputs=3
  Bus Selector : BusSelector  OutputSignals=GPS,y
  Bus Selector1 : BusSelector  OutputSignals=x_e,y_e,h_e
  Constant1 : Constant  Value=2
  Constant2 : Constant  Value=m
  Constant3 : Constant  Value=2
  Constant9 : Constant  Value=m
  Divide1 : Product  Inputs=*/
  Divide3 : Product  Inputs=*/
  Gain : Gain  Gain=-1
  Magnitude Squared : Math  Operator=magnitude^2
  Magnitude Squared1 : Math  Operator=magnitude^2
  Product1 : Product  Inputs=4
  Product2 : Product
  Product4 : Product  Inputs=4
  Product8 : Product
  Scope : Scope
  Selector : Selector  InputPortWidth=9  IndexOptions=Index vector (dialog)  Indices=1  OutputSizes=1
  Selector1 : Selector  InputPortWidth=9  IndexOptions=Index vector (dialog)  Indices=2  OutputSizes=1
  Selector2 : Selector  InputPortWidth=3  IndexOptions=Index vector (dialog)  Indices=1  OutputSizes=1
  Selector3 : Selector  InputPortWidth=3  IndexOptions=Index vector (dialog)  Indices=2  OutputSizes=1
  Selector4 : Selector  InputPortWidth=3  IndexOptions=Index vector (dialog)  Indices=2  OutputSizes=1
  Selector5 : Selector  InputPortWidth=3  IndexOptions=Index vector (dialog)  Indices=1  OutputSizes=1
  omega1 : Constant  Value=w1_out
  omega2 : Constant  Value=w2_out
  zeta1 : Constant  Value=zeta1_out
  zeta2 : Constant  Value=zeta2_out
  Outter Loop : Outport
  wires:
  Gain/1 -> Bus Creator/3  "Z_e"
  Bus Selector1/3 -> Gain/1  "<h_e>"
  Selector1/1 -> Product1/1  "y_dot"
  Product2/1 -> Add4/1
  Product8/1 -> Add/1
  Product1/1 -> Add4/2
  omega2/1 -> Product1/2, Magnitude Squared1/1
  Constant1/1 -> Product1/4
  Add2/1 -> Product2/1
  Add4/1 -> Bus Creator/2  "y_ddot"
  zeta2/1 -> Product1/3
  Magnitude Squared1/1 -> Product2/2
  Selector3/1 -> Add2/2  "y_e_measured"
  Selector2/1 -> Add1/2  "x_e_measured"
  Bus Selector/2 -> Selector/1, Selector1/1  "<y>"
  Bus Selector/1 -> Selector2/1, Selector3/1  "<GPS>"
  Bus Selector1/2 -> Add2/1  "<y_e>"
  Mission Planner/1 -> Bus Selector1/1
  Bus Creator/1 -> Outter Loop/1
  Magnitude Squared/1 -> Product8/2
  zeta1/1 -> Product4/3
  Add/1 -> Bus Creator/1, Scope/1  "x_ddot"
  Add1/1 -> Product8/1
  Constant3/1 -> Product4/4
  Bus Selector1/1 -> Add1/1  "<x_e>"
  omega1/1 -> Product4/2, Magnitude Squared/1
  Product4/1 -> Add/2
  Selector/1 -> Product4/1  "x_dot"
  Measured States/1 -> Bus Selector/1
  Divide3/1 -> Add4/3
  Constant9/1 -> Divide3/2
  Selector4/1 -> Divide3/1
  Divide1/1 -> Add/3
  Constant2/1 -> Divide1/2
  Selector5/1 -> Divide1/1
  Tension Force/1 -> Selector4/1, Selector5/1

== system Multi_Agent_Problem/Quadcopter2/Sensors ==
  X_e : Inport
  States : Inport  Port=2
  Bus Creator : BusCreator  Inputs=2
  Measured States : Outport
  wires:
  X_e/1 -> Bus Creator/1  "GPS"
  Bus Creator/1 -> Measured States/1
  States/1 -> Bus Creator/2  "y"
